simulink model "Pleiades"  (Simulink 10.0)
settings: Solver=ode45  StartTime=0.0  StopTime=3  RelTol=1e-3  EnableMultiTasking=on
settings Model: Creator=UX31  LastModifiedBy=unknown
settings DataIOCC: LimitDataPoints=on
settings DebuggingCC: UnderspecifiedInitializationDetection=Simplified  MergeDetectMultiDrivingBlocksExec=error  SolverPrmCheckMsg=warning
settings GRTTargetCC: GeneratePreprocessorConditionals=Disable all  CombineOutputUpdateFcns=on  GRTInterface=off
settings ConfigComp: CovExternalEMLEnable=off  CovSFcnEnable=off

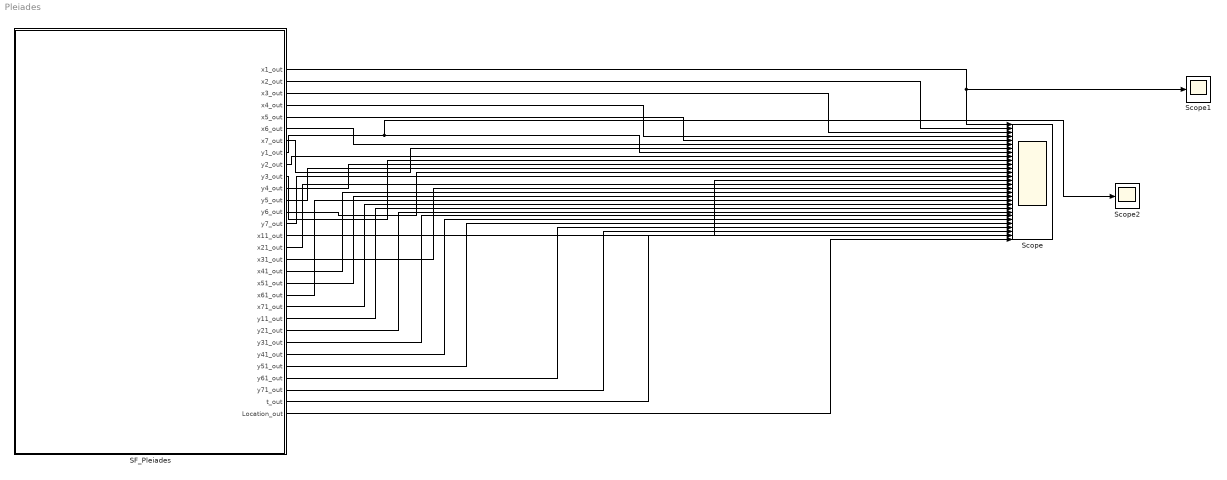
== system Pleiades ==
  SF_Pleiades : Stateflow chart  TreatAsAtomicUnit=on
  Scope : Scope  NumInputPorts=30
  Scope1 : Scope
  Scope2 : Scope
  wires:
  SF_Pleiades/1(x1_out) -> Scope/1, Scope1/1
  SF_Pleiades/2(x2_out) -> Scope/2
  SF_Pleiades/3(x3_out) -> Scope/3
  SF_Pleiades/4(x4_out) -> Scope/4
  SF_Pleiades/5(x5_out) -> Scope/5
  SF_Pleiades/6(x6_out) -> Scope/6
  SF_Pleiades/7(x7_out) -> Scope/7
  SF_Pleiades/9(y2_out) -> Scope/9
  SF_Pleiades/10(y3_out) -> Scope/10
  SF_Pleiades/11(y4_out) -> Scope/11
  SF_Pleiades/12(y5_out) -> Scope/12
  SF_Pleiades/13(y6_out) -> Scope/13
  SF_Pleiades/14(y7_out) -> Scope/14
  SF_Pleiades/15(x11_out) -> Scope/15
  SF_Pleiades/16(x21_out) -> Scope/16
  SF_Pleiades/17(x31_out) -> Scope/17
  SF_Pleiades/18(x41_out) -> Scope/18
  SF_Pleiades/19(x51_out) -> Scope/19
  SF_Pleiades/20(x61_out) -> Scope/20
  SF_Pleiades/21(x71_out) -> Scope/21
  SF_Pleiades/22(y11_out) -> Scope/22
  SF_Pleiades/23(y21_out) -> Scope/23
  SF_Pleiades/24(y31_out) -> Scope/24
  SF_Pleiades/25(y41_out) -> Scope/25
  SF_Pleiades/26(y51_out) -> Scope/26
  SF_Pleiades/27(y61_out) -> Scope/27
  SF_Pleiades/28(y71_out) -> Scope/28
  SF_Pleiades/29(t_out) -> Scope/29
  SF_Pleiades/30(Location_out) -> Scope/30
  SF_Pleiades/8(y1_out) -> Scope2/1, Scope/8

== stateflow chart SF_Pleiades ==
  settings: updateMethod=CONTINUOUS
  state Pleiades
    du:
    x1_dot = x11;
    x2_dot = x21;
    x3_dot = x31;
    x4_dot = x41;
    x5_dot = x51;
    x6_dot = x61;
    x7_dot = x71;
    y1_dot = y11;
    y2_dot = y21;
    y3_dot = y31;
    y4_dot = y41;
    y5_dot = y51;
    y6_dot = y61;
    y7_dot = y71;
    x11_dot = 2.0 * (x2 - x1) / ((x1 - x2) ^ 2.0 + (y1 - y2) ^ 2.0) ^ (3.0 / 2.0) + 3.0 * (x3 - x1) / ((x1 - x3) ^ 2.0 + (y1 - y3) ^ 2.0) ^ (3.0 / 2.0) + 4.0 * (x4 - x1) / ((x1 - x4) ^ 2.0 + (y1 - y4) ^ 2.0) ^ (3.0 / 2.0) + 5.0 * (x5 - x1) / ((x1 - x5) ^ 2.0 + (y1 - y5) ^ 2.0) ^ (3.0 / 2.0) + 6.0 * (x6 - x1) / ((x1 - x6) ^ 2.0 + (y1 - y6) ^ 2.0) ^ (3.0 / 2.0) + 7.0 * (x7 - x1) / ((x1 - x7) ^ 2.0 + (y1 - y7) ^ 2.0) ^ (3.0 / 2.0);
    x21_dot = 1.0 * (x1 - x2) / ((x1 - x2) ^ 2.0 + (y1 - y2) ^ 2.0) ^ (3.0 / 2.0) + 3.0 * (x3 - x2) / ((x2 - x3) ^ 2.0 + (y2 - y3) ^ 2.0) ^ (3.0 / 2.0) + 4.0 * (x4 - x2) / ((x2 - x4) ^ 2.0 + (y2 - y4) ^ 2.0) ^ (3.0 / 2.0) + 5.0 * (x5 - x2) / ((x2 - x5) ^ 2.0 + (y2 - y5) ^ 2.0) ^ (3.0 / 2.0) + 6.0 * (x6 - x2) / ((x2 - x6) ^ 2.0 + (y2 - y6) ^ 2.0) ^ (3.0 / 2.0) + 7.0 * (x7 - x2) / ((x2 - x7) ^ 2.0 + (y2 - y7) ^ 2.0) ^ (3.0 / 2.0);
    x31_dot = (2.0 * x2 - 2.0 * x3) / ((x2 - x3) ^ 2.0 + (y2 - y3) ^ 2.0) ^ (3.0 / 2.0) - (4.0 * x3 - 4.0 * x4) / ((x3 - x4) ^ 2.0 + (y3 - y4) ^ 2.0) ^ (3.0 / 2.0) - (5.0 * x3 - 5.0 * x5) / ((x3 - x5) ^ 2.0 + (y3 - y5) ^ 2.0) ^ (3.0 / 2.0) - (6.0 * x3 - 6.0 * x6) / ((x3 - x6) ^ 2.0 + (y3 - y6) ^ 2.0) ^ (3.0 / 2.0) - (7.0 * x3 - 7.0 * x7) / ((x3 - x7) ^ 2.0 + (y3 - y7) ^ 2.0) ^ (3.0 / 2.0) + (x1 - x3) / ((x1 - x3) ^ 2.0 + (y1 - y3) ^ 2.0) ^ (3.0 / 2.0);
    x41_dot = (2.0 * x2 - 2.0 * x4) / ((x2 - x4) ^ 2.0 + (y2 - y4) ^ 2.0) ^ (3.0 / 2.0) + (3.0 * x3 - 3.0 * x4) / ((x3 - x4) ^ 2.0 + (y3 - y4) ^ 2.0) ^ (3.0 / 2.0) - (5.0 * x4 - 5.0 * x5) / ((x4 - x5) ^ 2.0 + (y4 - y5) ^ 2.0) ^ (3.0 / 2.0) - (6.0 * x4 - 6.0 * x6) / ((x4 - x6) ^ 2.0 + (y4 - y6) ^ 2.0) ^ (3.0 / 2.0) - (7.0 * x4 - 7.0 * x7) / ((x4 - x7) ^ 2.0 + (y4 - y7) ^ 2.0) ^ (3.0 / 2.0) + (x1 - x4) / ((x1 - x4) ^ 2.0 + (y1 - y4) ^ 2.0) ^ (3.0 / 2.0);
    x51_dot = (2.0 * x2 - 2.0 * x5) / ((x2 - x5) ^ 2.0 + (y2 - y5) ^ 2.0) ^ (3.0 / 2.0) + (3.0 * x3 - 3.0 * x5) / ((x3 - x5) ^ 2.0 + (y3 - y5) ^ 2.0) ^ (3.0 / 2.0) + (4.0 * x4 - 4.0 * x5) / ((x4 - x5) ^ 2.0 + (y4 - y5) ^ 2.0) ^ (3.0 / 2.0) - (6.0 * x5 - 6.0 * x6) / ((x5 - x6) ^ 2.0 + (y5 - y6) ^ 2.0) ^ (3.0 / 2.0) - (7.0 * x5 - 7.0 * x7) / ((x5 - x7) ^ 2.0 + (y5 - y7) ^ 2.0) ^ (3.0 / 2.0) + (x1 - x5) / ((x1 - x5) ^ 2.0 + (y1 - y5) ^ 2.0) ^ (3.0 / 2.0);
    x61_dot = (2.0 * x2 - 2.0 * x6) / ((x2 - x6) ^ 2.0 + (y2 - y6) ^ 2.0) ^ (3.0 / 2.0) + (3.0 * x3 - 3.0 * x6) / ((x3 - x6) ^ 2.0 + (y3 - y6) ^ 2.0) ^ (3.0 / 2.0) + (4.0 * x4 - 4.0 * x6) / ((x4 - x6) ^ 2.0 + (y4 - y6) ^ 2.0) ^ (3.0 / 2.0) + (5.0 * x5 - 5.0 * x6) / ((x5 - x6) ^ 2.0 + (y5 - y6) ^ 2.0) ^ (3.0 / 2.0) - (7.0 * x6 - 7.0 * x7) / ((x6 - x7) ^ 2.0 + (y6 - y7) ^ 2.0) ^ (3.0 / 2.0) + (x1 - x6) / ((x1 - x6) ^ 2.0 + (y1 - y6) ^ 2.0) ^ (3.0 / 2.0);
    x71_dot = (2.0 * x2 - 2.0 * x7) / ((x2 - x7) ^ 2.0 + (y2 - y7) ^ 2.0) ^ (3.0 / 2.0) + (3.0 * x3 - 3.0 * x7) / ((x3 - x7) ^ 2.0 + (y3 - y7) ^ 2.0) ^ (3.0 / 2.0) + (4.0 * x4 - 4.0 * x7) / ((x4 - x7) ^ 2.0 + (y4 - y7) ^ 2.0) ^ (3.0 / 2.0) + (5.0 * x5 - 5.0 * x7) / ((x5 - x7) ^ 2.0 + (y5 - y7) ^ 2.0) ^ (3.0 / 2.0) + (6.0 * x6 - 6.0 * x7) / ((x6 - x7) ^ 2.0 + (y6 - y7) ^ 2.0) ^ (3.0 / 2.0) + (x1 - x7) / ((x1 - x7) ^ 2.0 + (y1 - y7) ^ 2.0) ^ (3.0 / 2.0);
    y11_dot = -(2.0 * y1 - 2.0 * y2) / ((x1 - x2) ^ 2.0 + (y1 - y2) ^ 2.0) ^ (3.0 / 2.0) - (3.0 * y1 - 3.0 * y3) / ((x1 - x3) ^ 2.0 + (y1 - y3) ^ 2.0) ^ (3.0 / 2.0) - (4.0 * y1 - 4.0 * y4) / ((x1 - x4) ^ 2.0 + (y1 - y4) ^ 2.0) ^ (3.0 / 2.0) - (5.0 * y1 - 5.0 * y5) / ((x1 - x5) ^ 2.0 + (y1 - y5) ^ 2.0) ^ (3.0 / 2.0) - (6.0 * y1 - 6.0 * y6) / ((x1 - x6) ^ 2.0 + (y1 - y6) ^ 2.0) ^ (3.0 / 2.0) - (7.0 * y1 - 7.0 * y7) / ((x1 - x7) ^ 2.0 + (y1 - y7) ^ 2.0) ^ (3.0 / 2.0);
    y21_dot = (y1 - y2) / ((x1 - x2) ^ 2.0 + (y1 - y2) ^ 2.0) ^ (3.0 / 2.0) - (4.0 * y2 - 4.0 * y4) / ((x2 - x4) ^ 2.0 + (y2 - y4) ^ 2.0) ^ (3.0 / 2.0) - (5.0 * y2 - 5.0 * y5) / ((x2 - x5) ^ 2.0 + (y2 - y5) ^ 2.0) ^ (3.0 / 2.0) - (6.0 * y2 - 6.0 * y6) / ((x2 - x6) ^ 2.0 + (y2 - y6) ^ 2.0) ^ (3.0 / 2.0) - (7.0 * y2 - 7.0 * y7) / ((x2 - x7) ^ 2.0 + (y2 - y7) ^ 2.0) ^ (3.0 / 2.0) - (3.0 * y2 - 3.0 * y3) / ((x2 - x3) ^ 2.0 + (y2 - y3) ^ 2.0) ^ (3.0 / 2.0);
    y31_dot = (2.0 * y2 - 2.0 * y3) / ((x2 - x3) ^ 2.0 + (y2 - y3) ^ 2.0) ^ (3.0 / 2.0) - (4.0 * y3 - 4.0 * y4) / ((x3 - x4) ^ 2.0 + (y3 - y4) ^ 2.0) ^ (3.0 / 2.0) - (5.0 * y3 - 5.0 * y5) / ((x3 - x5) ^ 2.0 + (y3 - y5) ^ 2.0) ^ (3.0 / 2.0) - (6.0 * y3 - 6.0 * y6) / ((x3 - x6) ^ 2.0 + (y3 - y6) ^ 2.0) ^ (3.0 / 2.0) - (7.0 * y3 - 7.0 * y7) / ((x3 - x7) ^ 2.0 + (y3 - y7) ^ 2.0) ^ (3.0 / 2.0) + (y1 - y3) / ((x1 - x3) ^ 2.0 + (y1 - y3) ^ 2.0) ^ (3.0 / 2.0);
    y41_dot = (2.0 * y2 - 2.0 * y4) / ((x2 - x4) ^ 2.0 + (y2 - y4) ^ 2.0) ^ (3.0 / 2.0) + (3.0 * y3 - 3.0 * y4) / ((x3 - x4) ^ 2.0 + (y3 - y4) ^ 2.0) ^ (3.0 / 2.0) - (5.0 * y4 - 5.0 * y5) / ((x4 - x5) ^ 2.0 + (y4 - y5) ^ 2.0) ^ (3.0 / 2.0) - (6.0 * y4 - 6.0 * y6) / ((x4 - x6) ^ 2.0 + (y4 - y6) ^ 2.0) ^ (3.0 / 2.0) - (7.0 * y4 - 7.0 * y7) / ((x4 - x7) ^ 2.0 + (y4 - y7) ^ 2.0) ^ (3.0 / 2.0) + (y1 - y4) / ((x1 - x4) ^ 2.0 + (y1 - y4) ^ 2.0) ^ (3.0 / 2.0);
    y51_dot = (2.0 * y2 - 2.0 * y5) / ((x2 - x5) ^ 2.0 + (y2 - y5) ^ 2.0) ^ (3.0 / 2.0) + (3.0 * y3 - 3.0 * y5) / ((x3 - x5) ^ 2.0 + (y3 - y5) ^ 2.0) ^ (3.0 / 2.0) + (4.0 * y4 - 4.0 * y5) / ((x4 - x5) ^ 2.0 + (y4 - y5) ^ 2.0) ^ (3.0 / 2.0) - (6.0 * y5 - 6.0 * y6) / ((x5 - x6) ^ 2.0 + (y5 - y6) ^ 2.0) ^ (3.0 / 2.0) - (7.0 * y5 - 7.0 * y7) / ((x5 - x7) ^ 2.0 + (y5 - y7) ^ 2.0) ^ (3.0 / 2.0) + (y1 - y5) / ((x1 - x5) ^ 2.0 + (y1 - y5) ^ 2.0) ^ (3.0 / 2.0);
    y61_dot = (2.0 * y2 - 2.0 * y6) / ((x2 - x6) ^ 2.0 + (y2 - y6) ^ 2.0) ^ (3.0 / 2.0) + (3.0 * y3 - 3.0 * y6) / ((x3 - x6) ^ 2.0 + (y3 - y6) ^ 2.0) ^ (3.0 / 2.0) + (4.0 * y4 - 4.0 * y6) / ((x4 - x6) ^ 2.0 + (y4 - y6) ^ 2.0) ^ (3.0 / 2.0) + (5.0 * y5 - 5.0 * y6) / ((x5 - x6) ^ 2.0 + (y5 - y6) ^ 2.0) ^ (3.0 / 2.0) - (7.0 * y6 - 7.0 * y7) / ((x6 - x7) ^ 2.0 + (y6 - y7) ^ 2.0) ^ (3.0 / 2.0) + (y1 - y6) / ((x1 - x6) ^ 2.0 + (y1 - y6) ^ 2.0) ^ (3.0 / 2.0);
    y71_dot = (2.0 * y2 - 2.0 * y7) / ((x2 - x7) ^ 2.0 + (y2 - y7) ^ 2.0) ^ (3.0 / 2.0) + (3.0 * y3 - 3.0 * y7) / ((x3 - x7) ^ 2.0 + (y3 - y7) ^ 2.0) ^ (3.0 / 2.0) + (4.0 * y4 - 4.0 * y7) / ((x4 - x7) ^ 2.0 + (y4 - y7) ^ 2.0) ^ (3.0 / 2.0) + (5.0 * y5 - 5.0 * y7) / ((x5 - x7) ^ 2.0 + (y5 - y7) ^ 2.0) ^ (3.0 / 2.0) + (6.0 * y6 - 6.0 * y7) / ((x6 - x7) ^ 2.0 + (y6 - y7) ^ 2.0) ^ (3.0 / 2.0) + (y1 - y7) / ((x1 - x7) ^ 2.0 + (y1 - y7) ^ 2.0) ^ (3.0 / 2.0);
    t_dot = 1.0;
    x1_out=x1;
    x2_out=x2;
    x3_out=x3;
    x4_out=x4;
    x5_out=x5;
    x6_out=x6;
    x7_out=x7;
    y1_out=y1;
    y2_out=y2;
    y3_out=y3;
    y4_out=y4;
    y5_out=y5;
    y6_out=y6;
    y7_out=y7;
    x11_out=x11;
    x21_out=x21;
    x31_out=x31;
    x41_out=x41;
    x51_out=x51;
    x61_out=x61;
    x71_out=x71;
    y11_out=y11;
    y21_out=y21;
    y31_out=y31;
    y41_out=y41;
    y51_out=y51;
    y61_out=y61;
    y71_out=y71;
    t_out=t;
    Location_out =1;
  (default) -> Pleiades : {t = 0.0; x1 = 3.0; x11 = 0.0; x2 = 3.0; x21 = 0.0; x3 = -1.0; x31 = 0.0; x4 = -3.0; x41 = 0.0; x5 = 2.0; x51 = 0.0; x6 = -2.0; x61 = 1.75; x7 = 2.0; x71 = -1.5; y1 = 3.0; y11 = 0.0; y2 = -3.0; y21 = 0.0; y3 = 2.0; y31 = 0.0; y4 = 0.0; y41 = -1.25; y5 = 0.0; y51 = 1.0; y6 = -4.0; y61 = 0.0; y7 = 4.0; y71 = 0.0;}
  data: stop_time constant double =2; x1 local double; x1_out output double; x2 local double; x2_out output double; x3 local double; x3_out output double; x4 local double; x4_out output double; x5 local double; x5_out output double; x6 local double; x6_out output double; x7 local double; x7_out output double; y1 local double; y1_out output double; y2 local double; y2_out output double; y3 local double; y3_out output double; y4 local double; y4_out output double; y5 local double; y5_out output double; y6 local double; y6_out output double; y7 local double; y7_out output double; x11 local double; x11_out output double; x21 local double; x21_out output double; x31 local double; x31_out output double; x41 local double; x41_out output double; x51 local double; x51_out output double; x61 local double; x61_out output double; x71 local double; x71_out output double; y11 local double; y11_out output double; y21 local double; y21_out output double; y31 local double; y31_out output double; y41 local double; y41_out output double; y51 local double; y51_out output double; y61 local double; y61_out output double; y71 local double; y71_out output double; t local double; t_out output double; Location_out output double
  data x1 settings: updateMethod=SF_CONTINUOUS_TIME_DATA
  data x2 settings: updateMethod=SF_CONTINUOUS_TIME_DATA
  data x3 settings: updateMethod=SF_CONTINUOUS_TIME_DATA
  data x4 settings: updateMethod=SF_CONTINUOUS_TIME_DATA
  data x5 settings: updateMethod=SF_CONTINUOUS_TIME_DATA
  data x6 settings: updateMethod=SF_CONTINUOUS_TIME_DATA
  data x7 settings: updateMethod=SF_CONTINUOUS_TIME_DATA
  data y1 settings: updateMethod=SF_CONTINUOUS_TIME_DATA
  data y2 settings: updateMethod=SF_CONTINUOUS_TIME_DATA
  data y3 settings: updateMethod=SF_CONTINUOUS_TIME_DATA
  data y4 settings: updateMethod=SF_CONTINUOUS_TIME_DATA
  data y5 settings: updateMethod=SF_CONTINUOUS_TIME_DATA
  data y6 settings: updateMethod=SF_CONTINUOUS_TIME_DATA
  data y7 settings: updateMethod=SF_CONTINUOUS_TIME_DATA
  data x11 settings: updateMethod=SF_CONTINUOUS_TIME_DATA
  data x21 settings: updateMethod=SF_CONTINUOUS_TIME_DATA
  data x31 settings: updateMethod=SF_CONTINUOUS_TIME_DATA
  data x41 settings: updateMethod=SF_CONTINUOUS_TIME_DATA
  data x51 settings: updateMethod=SF_CONTINUOUS_TIME_DATA
  data x61 settings: updateMethod=SF_CONTINUOUS_TIME_DATA
  data x71 settings: updateMethod=SF_CONTINUOUS_TIME_DATA
  data y11 settings: updateMethod=SF_CONTINUOUS_TIME_DATA
  data y21 settings: updateMethod=SF_CONTINUOUS_TIME_DATA
  data y31 settings: updateMethod=SF_CONTINUOUS_TIME_DATA
  data y41 settings: updateMethod=SF_CONTINUOUS_TIME_DATA
  data y51 settings: updateMethod=SF_CONTINUOUS_TIME_DATA
  data y61 settings: updateMethod=SF_CONTINUOUS_TIME_DATA
  data y71 settings: updateMethod=SF_CONTINUOUS_TIME_DATA
  data t settings: updateMethod=SF_CONTINUOUS_TIME_DATA
